simulink model "gm_PID_Discrete"  (R2021b)
settings: Solver=VariableStepAuto  StartTime=0.0  StopTime=10.0  RelTol=1e-3
libraries: slpidlib x1
settings Model: Creator=JelleKomen  LastModifiedBy=JelleKomen
settings OptimizationCC: BlockReduction=off  ConditionallyExecuteInputs=off
settings DebuggingCC: SignalRangeChecking=warning  InheritedTsInSrcMsg=none

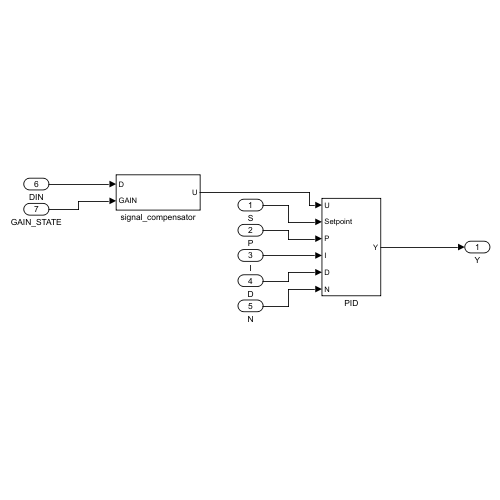
[thumbnail: Simulink's stored preview of the top-level diagram]
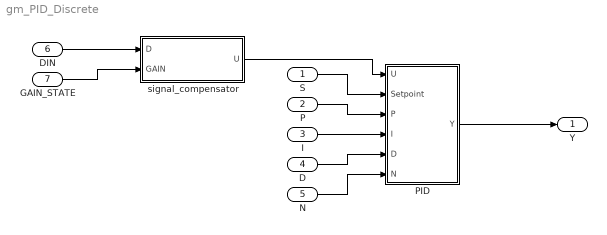
== system gm_PID_Discrete ==
  S : Inport  OutDataTypeStr=fixdt(1,32,24)
  P : Inport  Port=2  OutDataTypeStr=fixdt(1,32,24)
  I : Inport  Port=3  OutDataTypeStr=fixdt(1,32,24)
  D : Inport  Port=4  OutDataTypeStr=fixdt(1,32,24)
  N : Inport  Port=5  OutDataTypeStr=fixdt(1,32,24)
  DIN : Inport  Port=6  OutMin=-255  OutMax=256  OutDataTypeStr=fixdt(1,32,16)
  GAIN_STATE : Inport  Port=7  OutMin=0  OutMax=12  OutDataTypeStr=fixdt(1,8)
  PID : Subsystem
  signal_compensator : Subsystem
  Y : Outport  OutMin=-1023  OutMax=1024  OutDataTypeStr=fixdt(1,20)
  wires:
  GAIN_STATE/1 -> signal_compensator/2(GAIN)
  DIN/1 -> signal_compensator/1(D)
  signal_compensator/1(U) -> PID/1(U)
  N/1 -> PID/6(N)
  D/1 -> PID/5(D)
  I/1 -> PID/4(I)
  P/1 -> PID/3(P)
  S/1 -> PID/2(Setpoint)
  PID/1(Y) -> Y/1

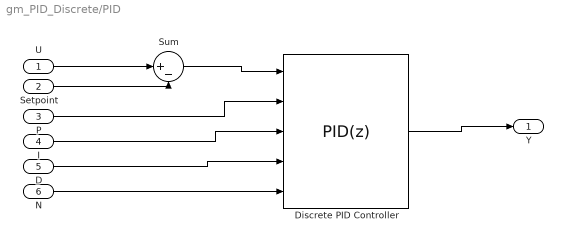
== system gm_PID_Discrete/PID ==
  U : Inport
  Setpoint : Inport  Port=2
  P : Inport  Port=3
  I : Inport  Port=4
  D : Inport  Port=5
  N : Inport  Port=6
  Discrete PID Controller : slpidlib/PID Controller  Controller=PID  Form=Parallel  TimeDomain=Discrete-time  UseExternalTs=off  SampleTime=-1  IntegratorMethod=Trapezoidal  FilterMethod=Forward Euler  ControllerParametersSource=external  P=1  I=1  D=0  UseFilter=on  N=100  TunerSelectOption=Transfer Function Based (PID Tuner App)  InitialConditionSource=internal  InitialConditionForIntegrator=0  InitialConditionForFilter=0  DifferentiatorICPrevScaledInput=0  ExternalReset=none  TrackingMode=off  Kt=1  LimitOutput=off  SatLimitsSource=internal  UpperSaturationLimit=inf  LowerSaturationLimit=-inf  LinearizeAsGain=off  AntiWindupMode=none  Kb=1  PGainOutDataTypeStr=fixdt(1,32,24)  PProdOutDataTypeStr=fixdt(1,32,24)  POutMin=[]  POutMax=[]  IGainOutDataTypeStr=fixdt(1,32,24)  IProdOutDataTypeStr=fixdt(1,32,24)  IOutMin=[]  IOutMax=[]  DGainOutDataTypeStr=fixdt(1,32,24)  DProdOutDataTypeStr=fixdt(1,32,24)  DOutMin=-126  DOutMax=127  NGainOutDataTypeStr=fixdt(1,32,24)  NProdOutDataTypeStr=fixdt(1,32,24)  NOutMin=[]  NOutMax=[]  SumOutDataTypeStr=fixdt(1,20)  SumOutMin=-1023  SumOutMax=1024  SaturationOutMin=[]  SaturationOutMax=[]  PParamMin=[]  PParamMax=[]  IParamMin=[]  IParamMax=[]  DParamMin=[]  DParamMax=[]  NParamMin=[]  NParamMax=[]  KbParamMin=[]  KbParamMax=[]  KtParamMin=[]  KtParamMax=[]  KbOutMin=[]  KbOutMax=[]  KtOutMin=[]  KtOutMax=[]  IntegratorOutMin=[]  IntegratorOutMax=[]  FilterOutMin=[]  FilterOutMax=[]  SumI1OutMin=[]  SumI1OutMax=[]  SumI2OutMin=[]  SumI2OutMax=[]  SumI3OutMin=[]  SumI3OutMax=[]  SumI4OutMin=[]  SumI4OutMax=[]  SumDOutMin=[]  SumDOutMax=[]  DifferentiatorOutMin=[]  DifferentiatorOutMax=[]  FilterDiffOutCoefMin=[]  FilterDiffOutCoefMax=[]  ReciprocalOutMin=[]  ReciprocalOutMax=[]  SumDenOutMin=[]  SumDenOutMax=[]  SumNumOutMin=[]  SumNumOutMax=[]  DivideOutMin=[]  DivideOutMax=[]  UdiffTsProdOutMin=[]  UdiffTsProdOutMax=[]  NTsProdOutMin=[]  NTsProdOutMax=[]  UintegralTsProdOutMin=[]  UintegralTsProdOutMax=[]  UngainTsProdOutMin=[]  UngainTsProdOutMax=[]  IntegratorContinuousStateAttributes=''  IntegratorStateMustResolveToSignalObject=off  IntegratorRTWStateStorageClass=Auto  FilterContinuousStateAttributes=''  FilterStateMustResolveToSignalObject=off  FilterRTWStateStorageClass=Auto  ParallelPVariant=ExternalParameters  IdealPVariant=Disabled  IVariant=ExternalParameters  DVariant=ExternalParameters  IntegratorVariant=Discrete  SatVariant=Disabled  AWVariant=Passthrough  PCopyVariant=Disabled  TRVariant=Disabled  FdbkBlocksVariant=Forward  IdealPFdbkVariant=Disabled  SatFdbkVariant=Disabled  DerivativeFilterVariant=ForwardEulerFilter  NVariant=ExternalParameters  NCopyVariant=Disabled  FilterICVariant=InternalICsFilter  IntegratorICVariant=InternalICs  ExternalResetVariant=Disabled  TRSumVariant=Passthrough  SumFdbkVariant=Disabled  SumVariant=Sum_PID  TsampFilterVariant=InternalTs  TsampNgainVariant=Passthrough  TsampIntegralVariant=Passthrough  ExternalSaturationOutDataTypeStr=Inherit: Same as second input
      settings: LockScale=on
  Sum : Sum  Inputs=|+-
  Y : Outport
  wires:
  Setpoint/1 -> Sum/2
  U/1 -> Sum/1
  Sum/1 -> Discrete PID Controller/1
  P/1 -> Discrete PID Controller/2
  N/1 -> Discrete PID Controller/5
  Discrete PID Controller/1 -> Y/1
  I/1 -> Discrete PID Controller/3
  D/1 -> Discrete PID Controller/4

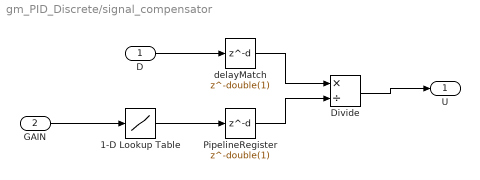
== system gm_PID_Discrete/signal_compensator ==
  D : Inport  OutMin=-32767  OutMax=32767  OutDataTypeStr=fixdt(1, 32, 16)  PortDimensions=1  SampleTime=1
  GAIN : Inport  Port=2  OutMin=0  OutMax=12  OutDataTypeStr=fixdt(1, 8, 3)  PortDimensions=1  SampleTime=1
  1-D Lookup Table : Lookup_n-D  NumberOfTableDimensions=1  BreakpointsForDimension1="fi(\"numerictype\",numerictype(1,8,3),\"fimath\",fimath(\"RoundingMethod\", \"Nearest\",\"OverflowAction\", \"Saturate\",\"ProductMode\",\"FullPrecision\",\"SumMode\",\"FullPrecision\"),\"Value\",\"[1 2 3 4 5 6 7 8 9 10 11 12]\")"  Table="reshape(fi(\"numerictype\",numerictype(1,20,8),\"fimath\",fimath(\"RoundingMethod\", \"Floor\",\"OverflowAction\", \"Wrap\",\"ProductMode\",\"FullPrecision\",\"SumMode\",\"FullPrecision\"),\"Value\",\"[0.125;0.15625;0.3125;0.625;1.25;2.5;5;10;20;40;80;160]\"), [1  12])"  InterpMethod=Flat  ExtrapMethod=Clip  DiagnosticForOutOfRangeInput=Error  SampleTime=1  OutDataTypeStr=fixdt(1, 20, 8)  RndMeth=Simplest  InputSameDT=on
  Divide : Product  Inputs=*/  OutDataTypeStr=fixdt(1, 24, 8)  RndMeth=Simplest  SaturateOnIntegerOverflow=on  SampleTime=1
  PipelineRegister : Delay  DelayLength=double(1)  InitialCondition=0  SampleTime=1
  delayMatch : Delay  DelayLength=double(1)  InitialCondition=0  SampleTime=1
  U : Outport  OutDataTypeStr=fixdt(1,24,8)  SampleTime=1
  wires:
  delayMatch/1 -> Divide/1
  GAIN/1 -> 1-D Lookup Table/1
  PipelineRegister/1 -> Divide/2
  Divide/1 -> U/1
  D/1 -> delayMatch/1
  1-D Lookup Table/1 -> PipelineRegister/1
